simulink model "TPCH2"  (Simulink 4.00)
settings: Solver=ode45  StartTime=0.0  StopTime=0.5  RelTol=1e-3
settings Model: BlockReductionOpt=off

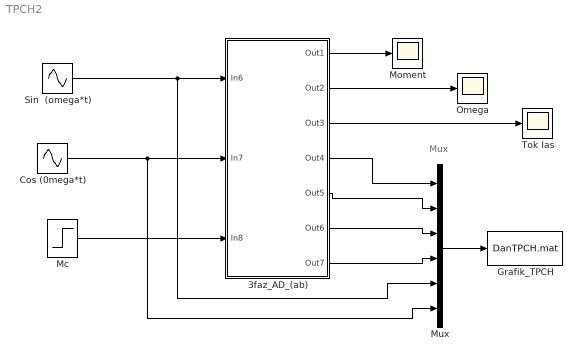
== system TPCH2 ==
  note: Mux
  " 3faz_AD_(ab)" : Subsystem
      settings: RTWFcnNameOpts=Auto  RTWFileNameOpts=Auto
  Cos (0mega*t) : Sin  Amplitude=311  Frequency=314  Phase=-pi/2  SampleTime=0
  Grafik_TPCH : ToFile  Filename=DanTPCH.mat  MatrixName=ans  SampleTime=-1
  Mc : Step  Time=0.06  Before=0.0  After=17  SampleTime=0
  Moment : Scope
      settings: TickLabels=on  TimeRange=80  YMin=-1  YMax=2  SaveToWorkspace=off  SaveName=ScopeData  DataFormat=Array  MaxDataPoints=5000
  Mux : Mux  Inputs=6
  Omega : Scope
      settings: TickLabels=on  TimeRange=0.5  YMin=0  YMax=200  SaveToWorkspace=off  DataFormat=Array  MaxDataPoints=5000
  Sin  (omega*t) : Sin  Amplitude=311  Frequency=314  Phase=0  SampleTime=0
  Tok Ias : Scope
      settings: TickLabels=on  TimeRange=0.5  YMin=-15  YMax=15  SaveToWorkspace=off  SaveName=ScopeData2  DataFormat=Array  MaxDataPoints=5000
  wires:
  " 3faz_AD_(ab)"/1(Out1) -> Moment/1
  " 3faz_AD_(ab)"/2(Out2) -> Omega/1
  " 3faz_AD_(ab)"/3(Out3) -> Tok Ias/1
  Cos (0mega*t)/1 -> " 3faz_AD_(ab)"/2(In7), Mux/6
  " 3faz_AD_(ab)"/4(Out4) -> Mux/1
  " 3faz_AD_(ab)"/5(Out5) -> Mux/2
  " 3faz_AD_(ab)"/6(Out6) -> Mux/3
  " 3faz_AD_(ab)"/7(Out7) -> Mux/4
  Mux/1 -> Grafik_TPCH/1
  Mc/1 -> " 3faz_AD_(ab)"/3(In8)
  Sin  (omega*t)/1 -> " 3faz_AD_(ab)"/1(In6), Mux/5

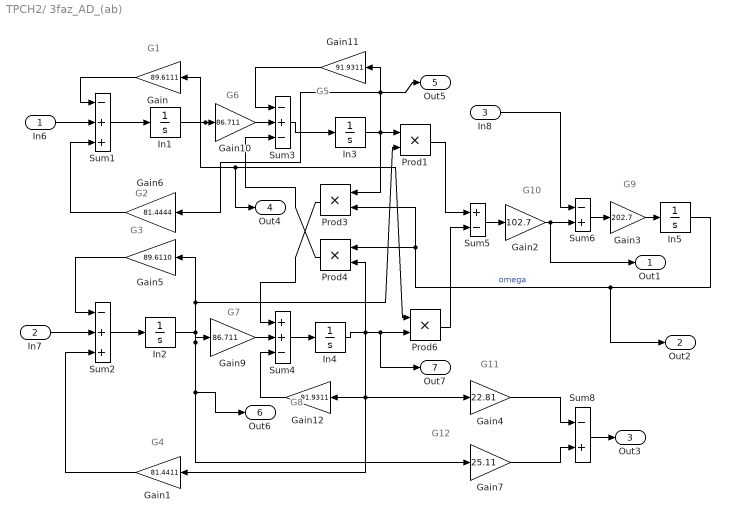
== system TPCH2/ 3faz_AD_(ab) ==
  note: G1
  note: G2
  note: G3
  note: G4
  note: G10
  note: G9
  note: G6
  note: G7
  note: G8
  note: G5
  note: G11
  note: G12
  In6 : Inport  Port=1
  In7 : Inport  Port=2
  In8 : Inport  Port=3
  "  Prod1" : Product  Inputs=2  Multiplication=Element-wise(.*)  SaturateOnIntegerOverflow=on
  Gain : Gain  Orientation=left  Gain=89.6111  Multiplication=Element-wise(K.*u)  SaturateOnIntegerOverflow=on
  Gain1 : Gain  Orientation=left  Gain=81.4411  Multiplication=Element-wise(K.*u)  SaturateOnIntegerOverflow=on
  Gain10 : Gain  Gain=86.711  Multiplication=Element-wise(K.*u)  SaturateOnIntegerOverflow=on
  Gain11 : Gain  Orientation=left  Gain=91.9311  Multiplication=Element-wise(K.*u)  SaturateOnIntegerOverflow=on
  Gain12 : Gain  Orientation=left  Gain=91.9311  Multiplication=Element-wise(K.*u)  SaturateOnIntegerOverflow=on
  Gain2 : Gain  Gain=102.7  Multiplication=Element-wise(K.*u)  SaturateOnIntegerOverflow=on
  Gain3 : Gain  Gain=202.7  Multiplication=Element-wise(K.*u)  SaturateOnIntegerOverflow=on
  Gain4 : Gain  Gain=22.81  Multiplication=Element-wise(K.*u)  SaturateOnIntegerOverflow=on
  Gain5 : Gain  Orientation=left  Gain=89.6110  Multiplication=Element-wise(K.*u)  SaturateOnIntegerOverflow=on
  Gain6 : Gain  Orientation=left  Gain=81.4444  Multiplication=Element-wise(K.*u)  SaturateOnIntegerOverflow=on
  Gain7 : Gain  Gain=25.11  Multiplication=Element-wise(K.*u)  SaturateOnIntegerOverflow=on
  Gain9 : Gain  Gain=86.711  Multiplication=Element-wise(K.*u)  SaturateOnIntegerOverflow=on
  In{1..5} (5 alike) : Integrator  ExternalReset=none  InitialConditionSource=internal  InitialCondition=0  LimitOutput=off  UpperSaturationLimit=inf  LowerSaturationLimit=-inf  ShowSaturationPort=off  ShowStatePort=off  AbsoluteTolerance=auto
  Prod3 : Product  Orientation=left  Inputs=2  Multiplication=Element-wise(.*)  SaturateOnIntegerOverflow=on
  Prod4 : Product  Orientation=left  Inputs=2  Multiplication=Element-wise(.*)  SaturateOnIntegerOverflow=on
  Prod6 : Product  Inputs=2  Multiplication=Element-wise(.*)  SaturateOnIntegerOverflow=on
  Sum1 : Sum  Inputs=-++  SaturateOnIntegerOverflow=on
  Sum2 : Sum  Inputs=-++  SaturateOnIntegerOverflow=on
  Sum3 : Sum  Inputs=-+-  SaturateOnIntegerOverflow=on
  Sum4 : Sum  Inputs=++-  SaturateOnIntegerOverflow=on
  Sum5 : Sum  Inputs=+-  SaturateOnIntegerOverflow=on
  Sum6 : Sum  Inputs=-+  SaturateOnIntegerOverflow=on
  Sum8 : Sum  Inputs=-+  SaturateOnIntegerOverflow=on
  Out1 : Outport  Port=1
  Out2 : Outport  Port=2
  Out3 : Outport  Port=3
  Out4 : Outport  Port=4
  Out5 : Outport  Port=5
  Out6 : Outport  Port=6
  Out7 : Outport  Port=7
  wires:
  Gain/1 -> Sum1/1
  Sum2/1 -> In2/1
  In4/1 -> Prod4/2, Gain1/1, Gain12/1, Gain4/1, Prod6/2, Out7/1
  In3/1 -> Prod3/1, "  Prod1"/1, Gain6/1, Gain11/1, Out5/1
  Prod6/1 -> Sum5/2
  Gain3/1 -> In5/1
  In8/1 -> Sum6/1
  "  Prod1"/1 -> Sum5/1
  Sum3/1 -> In3/1
  Sum5/1 -> Gain2/1
  Sum1/1 -> In1/1
  In2/1 -> "  Prod1"/2, Gain5/1, Gain9/1, Gain7/1, Out6/1
  In1/1 -> Gain10/1, Gain/1, Prod6/1, Out4/1
  Gain10/1 -> Sum3/2
  Gain9/1 -> Sum4/2
  Gain5/1 -> Sum2/1
  Prod4/1 -> Sum3/3
  Prod3/1 -> Sum4/1
  Gain2/1 -> Sum6/2, Out1/1
  Gain11/1 -> Sum3/1
  Gain12/1 -> Sum4/3
  In5/1 -> Prod3/2, Prod4/1, Out2/1  "omega"
  Sum4/1 -> In4/1
  Gain7/1 -> Sum8/2
  Gain4/1 -> Sum8/1
  Gain6/1 -> Sum1/3
  Gain1/1 -> Sum2/3
  In7/1 -> Sum2/2
  In6/1 -> Sum1/2
  Sum8/1 -> Out3/1
  Sum6/1 -> Gain3/1
